simulink model "Control_mod_sim"  (Simulink 8.9)
settings: Solver=ode45  StartTime=0.0  StopTime=tsim  MaxStep=1e-3  RelTol=1e-8  EnableMultiTasking=on
values from neighbouring files (symbols this model uses):
  N_Puntos = 10    [CONTROL_CINEMATICO.m]    (also in CONTROL_DINAMICO.m = 100)
  P_Fin = [-0.25; 0.05; 0.65]    [CONTROL_CINEMATICO.m]    (also in CONTROL_DINAMICO.m)
  P_Ini = [-0.1; 0.2; 0.5]    [CONTROL_CINEMATICO.m]    (also in CONTROL_DINAMICO.m)
  t_ini = 0.7    [CONTROL_CINEMATICO.m]    (also in CONTROL_DINAMICO.m = 3)
  t_mov = (N_Puntos + 2)*tsbc    (= 1.2)    [CONTROL_CINEMATICO.m]    (also in CONTROL_DINAMICO.m = 1.1)
settings Model: Creator=Manuel G. Ortega  LastModifiedBy=Javi Gómez  ExtModeTrigMode=oneshot  ExtModeArmWhenConnect=off
settings DataIOCC: LimitDataPoints=off
settings OptimizationCC: BooleanDataType=off  ExpressionDepthLimit=2147483647  InitFltsAndDblsToZero=on
settings DebuggingCC: SaveWithParameterizedLinksMsg=none  SignalResolutionControl=TryResolveAllWithWarning  MultiTaskDSMMsg=warning  MultiTaskCondExecSysMsg=none
settings HardwareCC: TargetUnknown=on
settings GRTTargetCC: TargetFcnLib=ansi_tfl_tmw.mat
settings ConfigComp: CovSFcnEnable=off

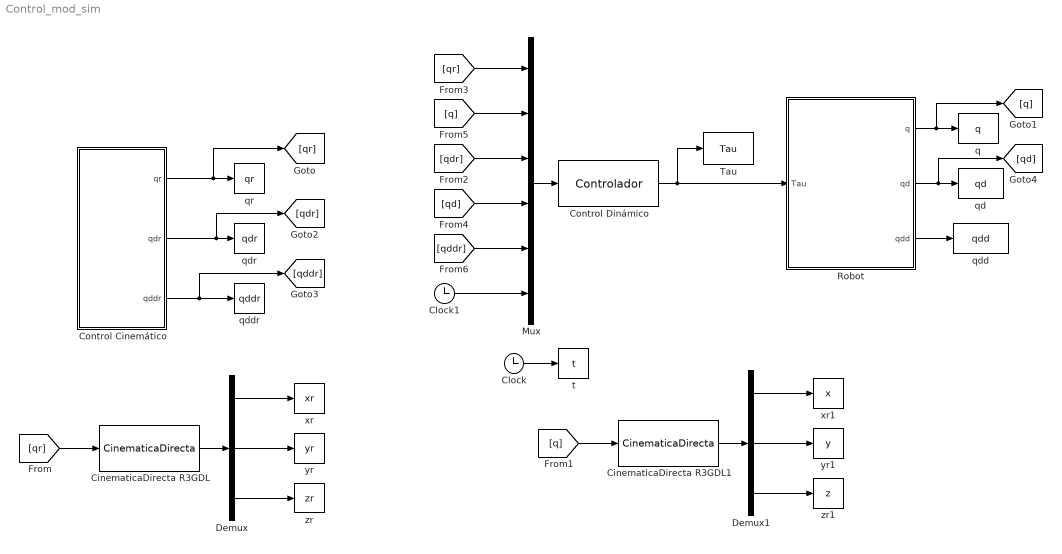
== system Control_mod_sim ==
  CinematicaDirecta R3GDL : MATLABFcn  MATLABFcn=CinematicaDirecta
  CinematicaDirecta R3GDL1 : MATLABFcn  MATLABFcn=CinematicaDirecta
  Clock : Clock
  Clock1 : Clock
  Control Cinemático : Subsystem
  Control Dinámico : MATLABFcn  MATLABFcn=Controlador  SampleTime=0.001
  Demux : Demux  Outputs=3
  Demux1 : Demux  Outputs=3
  Mux : Mux  Inputs=6
  Robot : Subsystem
  "Tau " : ToWorkspace  VariableName=Tau  SampleTime=-1
  q : ToWorkspace  VariableName=q  SampleTime=-1
  qd : ToWorkspace  VariableName=qd  SampleTime=-1
  qdd : ToWorkspace  VariableName=qdd  SampleTime=-1
  qddr : ToWorkspace  VariableName=qddr  SampleTime=-1
  qdr : ToWorkspace  VariableName=qdr  SampleTime=-1
  qr : ToWorkspace  VariableName=qr  SampleTime=-1
  t : ToWorkspace  VariableName=t  SampleTime=-1
  xr : ToWorkspace  VariableName=xr  SampleTime=-1
  xr1 : ToWorkspace  VariableName=x  SampleTime=-1
  yr : ToWorkspace  VariableName=yr  SampleTime=-1
  yr1 : ToWorkspace  VariableName=y  SampleTime=-1
  zr : ToWorkspace  VariableName=zr  SampleTime=-1
  zr1 : ToWorkspace  VariableName=z  SampleTime=-1
  wires:
  Clock/1 -> t/1
  [qr] -> CinematicaDirecta R3GDL/1
  CinematicaDirecta R3GDL/1 -> Demux/1
  Demux/1 -> xr/1
  Demux/2 -> yr/1
  Demux/3 -> zr/1
  Robot/3(qdd) -> qdd/1
  Control Dinámico/1 -> Robot/1(Tau), "Tau "/1
  Robot/2(qd) -> [qd], qd/1
  Robot/1(q) -> q/1, [q]
  Control Cinemático/1(qr) -> [qr], qr/1
  Control Cinemático/2(qdr) -> [qdr], qdr/1
  Control Cinemático/3(qddr) -> [qddr], qddr/1
  [qd] -> Mux/4
  Mux/1 -> Control Dinámico/1
  [q] -> Mux/2
  [qddr] -> Mux/5
  [qr] -> Mux/1
  Clock1/1 -> Mux/6
  [qdr] -> Mux/3
  [q] -> CinematicaDirecta R3GDL1/1
  Demux1/2 -> yr1/1
  Demux1/1 -> xr1/1
  CinematicaDirecta R3GDL1/1 -> Demux1/1
  Demux1/3 -> zr1/1

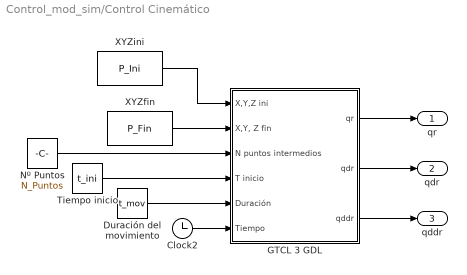
== system Control_mod_sim/Control Cinemático ==
  Clock2 : Clock
  Duración del movimiento : Constant  Value=t_mov
  GTCL 3 GDL : Subsystem
  Nº Puntos : Constant  Value=N_Puntos
  Tiempo inicio : Constant  Value=t_ini
  XYZfin : Constant  Value=P_Fin
  XYZini : Constant  Value=P_Ini
  qr : Outport
  qdr : Outport  Port=2
  qddr : Outport  Port=3
  wires:
  Duración del movimiento/1 -> GTCL 3 GDL/5(Duración)
  Tiempo inicio/1 -> GTCL 3 GDL/4(T inicio)
  XYZini/1 -> GTCL 3 GDL/1(X,Y,Z ini)
  GTCL 3 GDL/1(qr) -> qr/1
  XYZfin/1 -> GTCL 3 GDL/2("X,Y, Z fin")
  Nº Puntos/1 -> GTCL 3 GDL/3(N puntos intermedios)
  GTCL 3 GDL/2(qdr) -> qdr/1
  GTCL 3 GDL/3(qddr) -> qddr/1
  Clock2/1 -> GTCL 3 GDL/6(Tiempo)

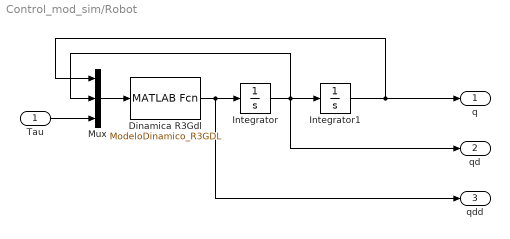
== system Control_mod_sim/Robot ==
  Tau : Inport
  Dinamica R3Gdl : MATLABFcn  MATLABFcn=ModeloDinamico_R3GDL
  Integrator : Integrator  InitialCondition=[0;0;0];
  Integrator1 : Integrator  InitialCondition=[0;0;0]
  Mux : Mux  Inputs=3
  q : Outport
  qd : Outport  Port=2
  qdd : Outport  Port=3
  wires:
  Mux/1 -> Dinamica R3Gdl/1
  Dinamica R3Gdl/1 -> Integrator/1, qdd/1
  Integrator/1 -> Integrator1/1, qd/1, Mux/2
  Integrator1/1 -> q/1, Mux/1
  Tau/1 -> Mux/3

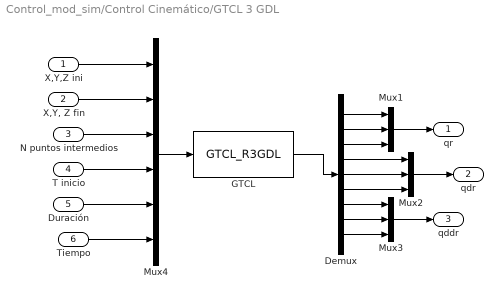
== system Control_mod_sim/Control Cinemático/GTCL 3 GDL ==
  X,Y,Z ini : Inport
  "X,Y, Z fin" : Inport  Port=2
  N puntos intermedios : Inport  Port=3
  T inicio : Inport  Port=4
  Duración : Inport  Port=5
  Tiempo : Inport  Port=6
  Demux : Demux  Outputs=9
  GTCL : MATLABFcn  MATLABFcn=GTCL_R3GDL  OutputDimensions=9
  Mux1 : Mux  Inputs=3
  Mux2 : Mux  Inputs=3
  Mux3 : Mux  Inputs=3
  Mux4 : Mux  Inputs=6
  qr : Outport
  qdr : Outport  Port=2
  qddr : Outport  Port=3
  wires:
  Mux1/1 -> qr/1
  Mux4/1 -> GTCL/1
  X,Y,Z ini/1 -> Mux4/1
  "X,Y, Z fin"/1 -> Mux4/2
  N puntos intermedios/1 -> Mux4/3
  T inicio/1 -> Mux4/4
  Duración/1 -> Mux4/5
  Tiempo/1 -> Mux4/6
  GTCL/1 -> Demux/1
  Demux/1 -> Mux1/1
  Demux/2 -> Mux1/2
  Demux/3 -> Mux1/3
  Mux2/1 -> qdr/1
  Demux/4 -> Mux2/1
  Demux/5 -> Mux2/2
  Demux/6 -> Mux2/3
  Mux3/1 -> qddr/1
  Demux/7 -> Mux3/1
  Demux/8 -> Mux3/2
  Demux/9 -> Mux3/3
